simulink subsystem "MotorEnergyLoss"  (R2023a)
settings: Solver=VariableStepAuto  StartTime=0.0  StopTime=10.0  RelTol=1e-3
settings Model: Creator=mrrom  LastModifiedBy=mrrom

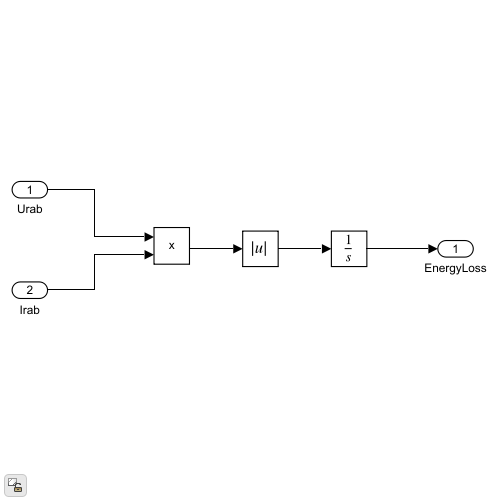
[thumbnail: Simulink's stored preview of the top-level diagram]
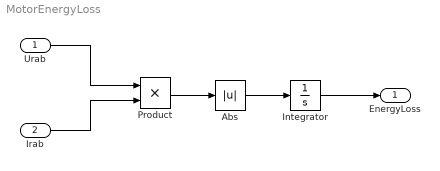
== system MotorEnergyLoss ==
  Urab : Inport
  Irab : Inport  Port=2
  Abs : Abs  SaturateOnIntegerOverflow=off
  Integrator : Integrator
  Product : Product
  EnergyLoss : Outport
  wires:
  Abs/1 -> Integrator/1
  Product/1 -> Abs/1
  Integrator/1 -> EnergyLoss/1
  Irab/1 -> Product/2
  Urab/1 -> Product/1
